simulink model "engine_model_211218"  (R2018b)
settings: Solver=VariableStepAuto  StartTime=0.0  StopTime=20  FixedStep=0.001  RelTol=1e-3
values from neighbouring files (symbols this model uses):
  F = 5e-5    (= 5e-05)    [BLDC_simulator.m]    (also in engine_parameters.m; engine_parameters_20191210.m = 1)
  J = 7.22e-6    (= 7.22e-06)    [BLDC_simulator.m]    (also in IMU.m = [cos(theta_2)*cos(theta_3) sin(theta_3) 0; engine_parameters.m; engine_parameters_20191210.m = 0.001)
  Kt = 8.44e-3    (= 0.00844)    [BLDC_simulator.m]    (also in engine_parameters.m)
  Kv = 8.44e-3    (= 0.00844)    [BLDC_simulator.m]    (also in engine_parameters.m)
  L = 0.42e-3    (= 0.00042)    [BLDC_simulator.m]    (also in engine_parameters.m; engine_parameters_20191210.m = 0.0005)
  R = 7.9    [BLDC_simulator.m]    (also in engine_parameters.m; engine_parameters_20191210.m = 0.5; inversekinematics.m = Rg*Rd*Rm)
undefined symbols (not defined in the file or in its folder): sigbuilder_block
libraries: simulink x7, simulink_extras x4
settings Model: Creator=Paweł Tymiński  LastModifiedBy=Paweł Tymiński

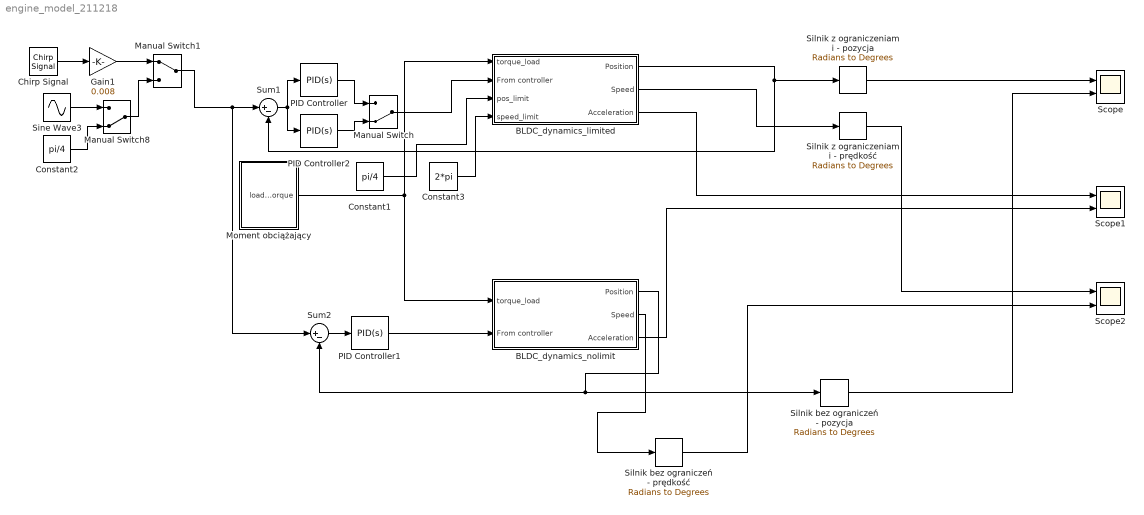
== system engine_model_211218 ==
  BLDC_dynamics_limited : Subsystem
  BLDC_dynamics_nolimit : Subsystem
  Chirp Signal : simulink/Sources/Chirp Signal  f1=1  T=20  f2=10
  Constant1 : Constant  Value=pi/4
  Constant2 : Constant  Value=pi/4
  Constant3 : Constant  Value=2*pi
  Gain1 : Gain  Gain=0.008
  Manual Switch : ManualSwitch  CurrentSetting=0
  Manual Switch1 : ManualSwitch
  Manual Switch8 : ManualSwitch  CurrentSetting=0
  Moment obciążający : Subsystem
  PID Controller : simulink/Continuous/PID Controller  Controller=PID  Form=Ideal  TimeDomain=Continuous-time  SampleTime=-1  IntegratorMethod=Forward Euler  FilterMethod=Forward Euler  ControllerParametersSource=internal  P=3.75221520248844  I=9.20583270553454  D=0.233305479962469  UseFilter=on  N=39454.8430256031  TunerSelectOption=Transfer Function Based (PID Tuner App)  InitialConditionSource=internal  InitialConditionForIntegrator=0  InitialConditionForFilter=0  DifferentiatorICPrevScaledInput=0  ExternalReset=none  TrackingMode=off  Kt=1  LimitOutput=off  UpperSaturationLimit=inf  LowerSaturationLimit=-inf  LinearizeAsGain=on  AntiWindupMode=none  Kb=1  POutMin=[]  POutMax=[]  IOutMin=[]  IOutMax=[]  DOutMin=[]  DOutMax=[]  NOutMin=[]  NOutMax=[]  SumOutMin=[]  SumOutMax=[]  SaturationOutMin=[]  SaturationOutMax=[]  PParamMin=[]  PParamMax=[]  IParamMin=[]  IParamMax=[]  DParamMin=[]  DParamMax=[]  NParamMin=[]  NParamMax=[]  KbParamMin=[]  KbParamMax=[]  KtParamMin=[]  KtParamMax=[]  KbOutMin=[]  KbOutMax=[]  KtOutMin=[]  KtOutMax=[]  IntegratorOutMin=[]  IntegratorOutMax=[]  FilterOutMin=[]  FilterOutMax=[]  SumI1OutMin=[]  SumI1OutMax=[]  SumI2OutMin=[]  SumI2OutMax=[]  SumI3OutMin=[]  SumI3OutMax=[]  SumI4OutMin=[]  SumI4OutMax=[]  SumDOutMin=[]  SumDOutMax=[]  DifferentiatorOutMin=[]  DifferentiatorOutMax=[]  FilterDiffOutCoefMin=[]  FilterDiffOutCoefMax=[]  ReciprocalOutMin=[]  ReciprocalOutMax=[]  SumDenOutMin=[]  SumDenOutMax=[]  SumNumOutMin=[]  SumNumOutMax=[]  DivideOutMin=[]  DivideOutMax=[]  IntegratorContinuousStateAttributes=''  IntegratorStateMustResolveToSignalObject=off  IntegratorRTWStateStorageClass=Auto  FilterContinuousStateAttributes=''  FilterStateMustResolveToSignalObject=off  FilterRTWStateStorageClass=Auto  ParallelPVariant=Passthrough  IdealPVariant=InternalParameters  IVariant=InternalParameters  DVariant=InternalParameters  IntegratorVariant=Continuous  SatVariant=Disabled  AWVariant=Passthrough  PCopyVariant=Disabled  TRVariant=Disabled  FdbkBlocksVariant=Forward  IdealPFdbkVariant=Disabled  SatFdbkVariant=Disabled  DerivativeFilterVariant=ContFilter  NVariant=InternalParameters  NCopyVariant=Disabled  FilterICVariant=InternalICsFilter  IntegratorICVariant=InternalICs  ExternalResetVariant=Disabled  TRSumVariant=Passthrough  SumFdbkVariant=Disabled  SumVariant=Sum_PID
  PID Controller1 : simulink/Continuous/PID Controller  Controller=PID  Form=Ideal  TimeDomain=Continuous-time  SampleTime=-1  IntegratorMethod=Forward Euler  FilterMethod=Forward Euler  ControllerParametersSource=internal  P=5.17125627242477  I=0.879628779481434  D=0.157743378330372  UseFilter=on  N=13783.089028979  TunerSelectOption=Transfer Function Based (PID Tuner App)  InitialConditionSource=internal  InitialConditionForIntegrator=0  InitialConditionForFilter=0  DifferentiatorICPrevScaledInput=0  ExternalReset=none  TrackingMode=off  Kt=1  LimitOutput=off  UpperSaturationLimit=inf  LowerSaturationLimit=-inf  LinearizeAsGain=on  AntiWindupMode=none  Kb=1  POutMin=[]  POutMax=[]  IOutMin=[]  IOutMax=[]  DOutMin=[]  DOutMax=[]  NOutMin=[]  NOutMax=[]  SumOutMin=[]  SumOutMax=[]  SaturationOutMin=[]  SaturationOutMax=[]  PParamMin=[]  PParamMax=[]  IParamMin=[]  IParamMax=[]  DParamMin=[]  DParamMax=[]  NParamMin=[]  NParamMax=[]  KbParamMin=[]  KbParamMax=[]  KtParamMin=[]  KtParamMax=[]  KbOutMin=[]  KbOutMax=[]  KtOutMin=[]  KtOutMax=[]  IntegratorOutMin=[]  IntegratorOutMax=[]  FilterOutMin=[]  FilterOutMax=[]  SumI1OutMin=[]  SumI1OutMax=[]  SumI2OutMin=[]  SumI2OutMax=[]  SumI3OutMin=[]  SumI3OutMax=[]  SumI4OutMin=[]  SumI4OutMax=[]  SumDOutMin=[]  SumDOutMax=[]  DifferentiatorOutMin=[]  DifferentiatorOutMax=[]  FilterDiffOutCoefMin=[]  FilterDiffOutCoefMax=[]  ReciprocalOutMin=[]  ReciprocalOutMax=[]  SumDenOutMin=[]  SumDenOutMax=[]  SumNumOutMin=[]  SumNumOutMax=[]  DivideOutMin=[]  DivideOutMax=[]  IntegratorContinuousStateAttributes=''  IntegratorStateMustResolveToSignalObject=off  IntegratorRTWStateStorageClass=Auto  FilterContinuousStateAttributes=''  FilterStateMustResolveToSignalObject=off  FilterRTWStateStorageClass=Auto  ParallelPVariant=Passthrough  IdealPVariant=InternalParameters  IVariant=InternalParameters  DVariant=InternalParameters  IntegratorVariant=Continuous  SatVariant=Disabled  AWVariant=Passthrough  PCopyVariant=Disabled  TRVariant=Disabled  FdbkBlocksVariant=Forward  IdealPFdbkVariant=Disabled  SatFdbkVariant=Disabled  DerivativeFilterVariant=ContFilter  NVariant=InternalParameters  NCopyVariant=Disabled  FilterICVariant=InternalICsFilter  IntegratorICVariant=InternalICs  ExternalResetVariant=Disabled  TRSumVariant=Passthrough  SumFdbkVariant=Disabled  SumVariant=Sum_PID
  PID Controller2 : simulink/Continuous/PID Controller  Controller=PID  Form=Ideal  TimeDomain=Continuous-time  SampleTime=-1  IntegratorMethod=Forward Euler  FilterMethod=Forward Euler  ControllerParametersSource=internal  P=5.17125627242477  I=0.879628779481434  D=0.157743378330372  UseFilter=on  N=13783.089028979  TunerSelectOption=Transfer Function Based (PID Tuner App)  InitialConditionSource=internal  InitialConditionForIntegrator=0  InitialConditionForFilter=0  DifferentiatorICPrevScaledInput=0  ExternalReset=none  TrackingMode=off  Kt=1  LimitOutput=off  UpperSaturationLimit=inf  LowerSaturationLimit=-inf  LinearizeAsGain=on  AntiWindupMode=none  Kb=1  POutMin=[]  POutMax=[]  IOutMin=[]  IOutMax=[]  DOutMin=[]  DOutMax=[]  NOutMin=[]  NOutMax=[]  SumOutMin=[]  SumOutMax=[]  SaturationOutMin=[]  SaturationOutMax=[]  PParamMin=[]  PParamMax=[]  IParamMin=[]  IParamMax=[]  DParamMin=[]  DParamMax=[]  NParamMin=[]  NParamMax=[]  KbParamMin=[]  KbParamMax=[]  KtParamMin=[]  KtParamMax=[]  KbOutMin=[]  KbOutMax=[]  KtOutMin=[]  KtOutMax=[]  IntegratorOutMin=[]  IntegratorOutMax=[]  FilterOutMin=[]  FilterOutMax=[]  SumI1OutMin=[]  SumI1OutMax=[]  SumI2OutMin=[]  SumI2OutMax=[]  SumI3OutMin=[]  SumI3OutMax=[]  SumI4OutMin=[]  SumI4OutMax=[]  SumDOutMin=[]  SumDOutMax=[]  DifferentiatorOutMin=[]  DifferentiatorOutMax=[]  FilterDiffOutCoefMin=[]  FilterDiffOutCoefMax=[]  ReciprocalOutMin=[]  ReciprocalOutMax=[]  SumDenOutMin=[]  SumDenOutMax=[]  SumNumOutMin=[]  SumNumOutMax=[]  DivideOutMin=[]  DivideOutMax=[]  IntegratorContinuousStateAttributes=''  IntegratorStateMustResolveToSignalObject=off  IntegratorRTWStateStorageClass=Auto  FilterContinuousStateAttributes=''  FilterStateMustResolveToSignalObject=off  FilterRTWStateStorageClass=Auto  ParallelPVariant=Passthrough  IdealPVariant=InternalParameters  IVariant=InternalParameters  DVariant=InternalParameters  IntegratorVariant=Continuous  SatVariant=Disabled  AWVariant=Passthrough  PCopyVariant=Disabled  TRVariant=Disabled  FdbkBlocksVariant=Forward  IdealPFdbkVariant=Disabled  SatFdbkVariant=Disabled  DerivativeFilterVariant=ContFilter  NVariant=InternalParameters  NCopyVariant=Disabled  FilterICVariant=InternalICsFilter  IntegratorICVariant=InternalICs  ExternalResetVariant=Disabled  TRSumVariant=Passthrough  SumFdbkVariant=Disabled  SumVariant=Sum_PID
  Scope : Scope  NumInputPorts=2
  Scope1 : Scope  NumInputPorts=2
  Scope2 : Scope  NumInputPorts=2
  Silnik bez ograniczeń - pozycja : simulink_extras/Transformations/Radians to Degrees
  Silnik bez ograniczeń - prędkość : simulink_extras/Transformations/Radians to Degrees
  Silnik z ograniczeniami - pozycja : simulink_extras/Transformations/Radians to Degrees
  Silnik z ograniczeniami - prędkość : simulink_extras/Transformations/Radians to Degrees
  Sine Wave3 : Sin  Amplitude=pi/18  Frequency=2*pi  SampleTime=0
  Sum1 : Sum  Inputs=|+-
  Sum2 : Sum  Inputs=|+-
  wires:
  Sum1/1 -> PID Controller2/1, PID Controller/1
  Manual Switch1/1 -> Sum1/1, Sum2/1
  Moment obciążający/1(load_torque) -> BLDC_dynamics_nolimit/1(torque_load), BLDC_dynamics_limited/1(torque_load)
  Constant1/1 -> BLDC_dynamics_limited/3(pos_limit)
  BLDC_dynamics_limited/1(Position) -> Silnik z ograniczeniami - pozycja/1, Sum1/2
  BLDC_dynamics_limited/2(Speed) -> Silnik z ograniczeniami - prędkość/1
  Silnik z ograniczeniami - pozycja/1 -> Scope/1
  Sum2/1 -> PID Controller1/1
  PID Controller1/1 -> BLDC_dynamics_nolimit/2(From controller)
  BLDC_dynamics_nolimit/1(Position) -> Sum2/2, Silnik bez ograniczeń - pozycja/1
  BLDC_dynamics_nolimit/2(Speed) -> Silnik bez ograniczeń - prędkość/1
  Silnik bez ograniczeń - pozycja/1 -> Scope/2
  Silnik bez ograniczeń - prędkość/1 -> Scope2/2
  Manual Switch/1 -> BLDC_dynamics_limited/2(From controller)
  PID Controller/1 -> Manual Switch/1
  PID Controller2/1 -> Manual Switch/2
  Silnik z ograniczeniami - prędkość/1 -> Scope2/1
  Constant3/1 -> BLDC_dynamics_limited/4(speed_limit)
  BLDC_dynamics_nolimit/3(Acceleration) -> Scope1/2
  BLDC_dynamics_limited/3(Acceleration) -> Scope1/1
  Sine Wave3/1 -> Manual Switch8/1
  Constant2/1 -> Manual Switch8/2
  Chirp Signal/1 -> Gain1/1
  Manual Switch8/1 -> Manual Switch1/2
  Gain1/1 -> Manual Switch1/1

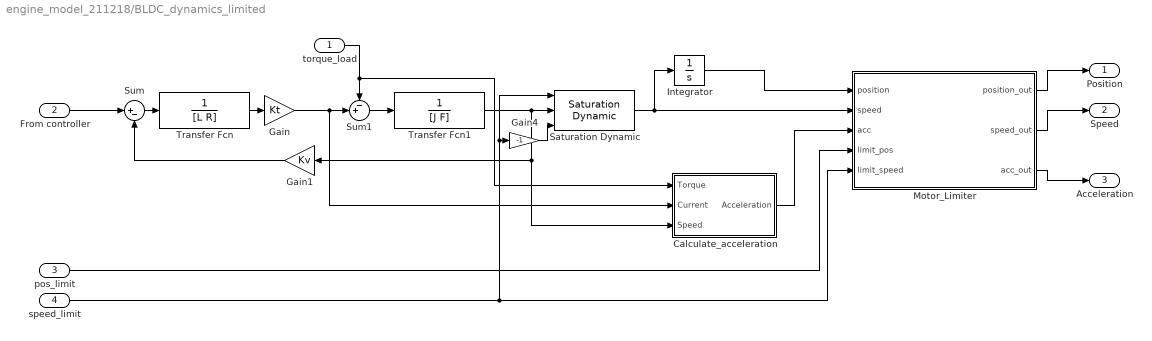
== system engine_model_211218/BLDC_dynamics_limited ==
  torque_load : Inport
  From controller : Inport  Port=2
  pos_limit : Inport  Port=3
  speed_limit : Inport  Port=4
  Calculate_acceleration : Subsystem
  Gain : Gain  Gain=Kt
  Gain1 : Gain  Gain=Kv
  Gain4 : Gain  Gain=-1
  Integrator : Integrator
  Motor_Limiter : MATLAB Function  TreatAsAtomicUnit=on
  Saturation Dynamic : simulink/Discontinuities/Saturation Dynamic  OutMin=[]  OutMax=[]  OutDataTypeStr=Inherit: Same as second input  OutDataType=fixdt(1, 16)  OutScaling=2^-10  DoSatur=off
  Sum : Sum  Inputs=|+-
  Sum1 : Sum  Inputs=-+|
  Transfer Fcn : TransferFcn  Denominator=[L R]
  Transfer Fcn1 : TransferFcn  Denominator=[J F]
  Position : Outport
  Speed : Outport  Port=2
  Acceleration : Outport  Port=3
  wires:
  Gain/1 -> Calculate_acceleration/2(Current), Sum1/2
  Transfer Fcn/1 -> Gain/1
  Sum/1 -> Transfer Fcn/1
  From controller/1 -> Sum/1
  torque_load/1 -> Calculate_acceleration/1(Torque), Sum1/1
  Gain1/1 -> Sum/2
  Sum1/1 -> Transfer Fcn1/1
  Transfer Fcn1/1 -> Calculate_acceleration/3(Speed), Gain1/1, Saturation Dynamic/2
  Saturation Dynamic/1 -> Motor_Limiter/2(speed), Integrator/1
  Gain4/1 -> Saturation Dynamic/3
  Motor_Limiter/1(position_out) -> Position/1
  Motor_Limiter/2(speed_out) -> Speed/1
  Motor_Limiter/3(acc_out) -> Acceleration/1
  Calculate_acceleration/1(Acceleration) -> Motor_Limiter/3(acc)
  Integrator/1 -> Motor_Limiter/1(position)
  speed_limit/1 -> Saturation Dynamic/1, Gain4/1, Motor_Limiter/5(limit_speed)
  pos_limit/1 -> Motor_Limiter/4(limit_pos)

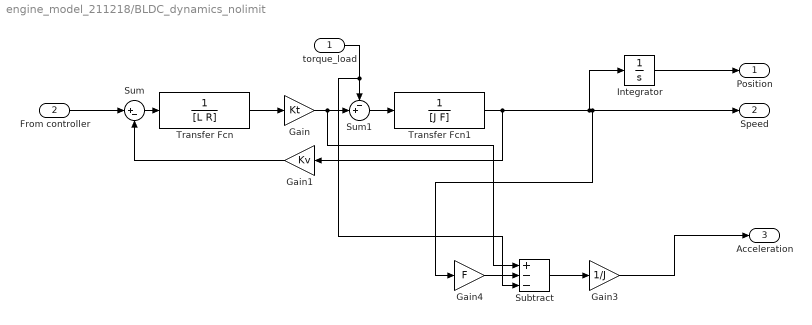
== system engine_model_211218/BLDC_dynamics_nolimit ==
  torque_load : Inport
  From controller : Inport  Port=2
  Gain : Gain  Gain=Kt
  Gain1 : Gain  Gain=Kv
  Gain3 : Gain  Gain=1/J
  Gain4 : Gain  Gain=F
  Integrator : Integrator
  Subtract : Sum  Inputs=+--
  Sum : Sum  Inputs=|+-
  Sum1 : Sum  Inputs=-+|
  Transfer Fcn : TransferFcn  Denominator=[L R]
  Transfer Fcn1 : TransferFcn  Denominator=[J F]
  Position : Outport
  Speed : Outport  Port=2
  Acceleration : Outport  Port=3
  wires:
  Transfer Fcn/1 -> Gain/1
  Sum/1 -> Transfer Fcn/1
  From controller/1 -> Sum/1
  Gain1/1 -> Sum/2
  Sum1/1 -> Transfer Fcn1/1
  Integrator/1 -> Position/1
  Subtract/1 -> Gain3/1
  Gain4/1 -> Subtract/2
  Gain3/1 -> Acceleration/1
  Gain/1 -> Subtract/1, Sum1/2
  torque_load/1 -> Subtract/3, Sum1/1
  Transfer Fcn1/1 -> Integrator/1, Gain4/1, Speed/1, Gain1/1

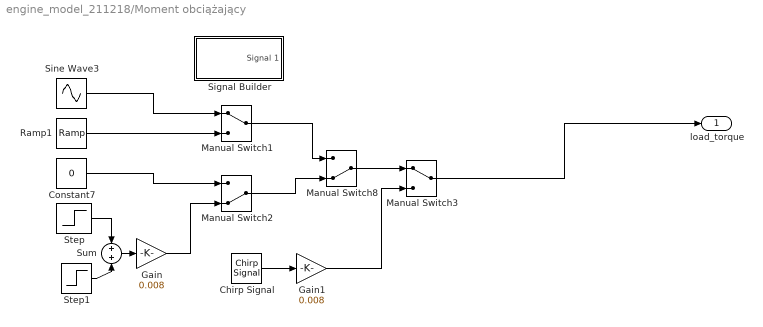
== system engine_model_211218/Moment obciążający ==
  Chirp Signal : simulink/Sources/Chirp Signal  f1=1  T=20  f2=10
  Constant7 : Constant  Value=0
  Gain : Gain  Gain=0.008
  Gain1 : Gain  Gain=0.008
  Manual Switch1 : ManualSwitch
  Manual Switch2 : ManualSwitch  CurrentSetting=0
  Manual Switch3 : ManualSwitch
  Manual Switch8 : ManualSwitch  CurrentSetting=0
  Ramp1 : simulink/Sources/Ramp  slope=pi/16  start=0  InitialOutput=0
  Signal Builder : Subsystem  Tag=STV Subsys  LoadFcn=sigbuilder_block('load');  StartFcn=sigbuilder_block('start');  StopFcn=sigbuilder_block('stop');  ClipboardFcn=sigbuilder_block('clipboard');  mask(Sigbuilder block){tuvar=[0:10]}
      mask help: Simulink:masks:SigbuilderBlock_MD
      mask init:
      | if ~strcmp(get_param(bdroot(gcbh),'SimulationStatus'),'stopped') tuvar = sigbuilder_block('maskInit'); end
      settings: CopyFcn=sigbuilder_block('copy');  DeleteFcn=sigbuilder_block('delete');  ModelCloseFcn=sigbuilder_block('modelClose');  PreSaveFcn=sigbuilder_block('preSave');  PauseFcn=sigbuilder_block('pause');  ContinueFcn=sigbuilder_block('continue');  NameChangeFcn=sigbuilder_block('namechange');  OpenFcn=sigbuilder_block('open',[437.6 199.2 550.4 400 ]);  CloseFcn=sigbuilder_block('close');
      mask Display: plot(0, 0, 100, 100,[2, 2, 32, 32, 2], [68, 8, 8, 68, 68],[32, 2], [38, 38], [32, 19, 2],[53, 60, 44], [32, 17, 17, 2],[16, 16, 31, 31]);txt = getActiveGroup(gcbh);text(2, 100, txt,'verticalAlignment', 'top');
  Sine Wave3 : Sin  Amplitude=pi/18  SampleTime=0
  Step : Step  SampleTime=0
  Step1 : Step  Time=2  After=-1  SampleTime=0
  Sum : Sum
  load_torque : Outport
  wires:
  Step/1 -> Sum/1
  Constant7/1 -> Manual Switch2/1
  Gain/1 -> Manual Switch2/2
  Step1/1 -> Sum/2
  Sine Wave3/1 -> Manual Switch1/1
  Manual Switch1/1 -> Manual Switch8/1
  Manual Switch2/1 -> Manual Switch8/2
  Sum/1 -> Gain/1
  Ramp1/1 -> Manual Switch1/2
  Chirp Signal/1 -> Gain1/1
  Manual Switch3/1 -> load_torque/1
  Manual Switch8/1 -> Manual Switch3/1
  Gain1/1 -> Manual Switch3/2

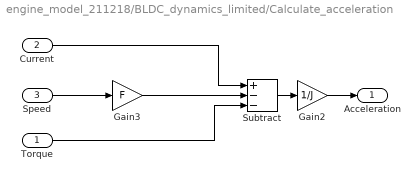
== system engine_model_211218/BLDC_dynamics_limited/Calculate_acceleration ==
  Torque : Inport
  Current : Inport  Port=2
  Speed : Inport  Port=3
  Gain2 : Gain  Gain=1/J
  Gain3 : Gain  Gain=F
  Subtract : Sum  Inputs=+--
  Acceleration : Outport
  wires:
  Gain3/1 -> Subtract/2
  Subtract/1 -> Gain2/1
  Gain2/1 -> Acceleration/1
  Current/1 -> Subtract/1
  Speed/1 -> Gain3/1
  Torque/1 -> Subtract/3

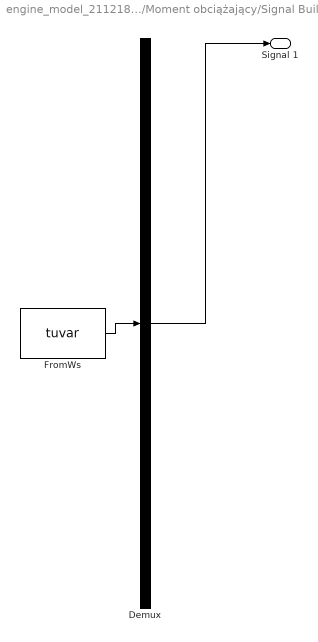
== system engine_model_211218/Moment obciążający/Signal Builder ==
  Demux : Demux  Tag=STV Demux  Outputs=1
  FromWs : FromWorkspace  Tag=STV FromWs  VariableName=tuvar  SampleTime=0
      SigBuilderData=|
      | common.afterFinalStr = 'Extrapolate'
      | common.sampleTime = 0
      | dataSet.timeRange = [0 10]
      | dataSet.name = 'Group 1'
      | sbobj.Groups.Name = 'Group 1'
      | sbobj.Groups.Signals.Name = 'Signal 1'
      | sbobj.Groups.Signals.XData = [0 4 4 6 6 10]
      | sbobj.Groups.Signals.YData = [-0.015 0.125 0.575 0.895 0.04 0]
  Signal 1 : Outport  Tag=STV Outport
  wires:
  Demux/1 -> Signal 1/1
  FromWs/1 -> Demux/1

== matlab function engine_model_211218/BLDC_dynamics_limited/Motor_Limiter ==
  data: position input; position_out output; speed input; speed_out output; acc input; limit_pos input; limit_speed input; acc_out output
function [position_out,speed_out,acc_out] = fcn(position, speed,  acc, limit_pos, limit_speed)

if abs(position)<=limit_pos        
    position_out=position;
    speed_out=speed;
else
    position_out=sign(position)*limit_pos;   
    speed_out=0;
end

if abs(speed)<=limit_speed & abs(position)<=limit_pos
    acc_out=acc;
else
    acc_out=0;
end
